simulink subsystem "RT_BladeElementForces"  (R2025a)
settings: Solver=VariableStepAuto  StartTime=0.0  StopTime=10.0  RelTol=1e-3
undefined symbols (not defined in the file): RT_AirDensity_P, RT_BEDistFromEffSta_A, RT_NondimRadialDisRef_P, RT_NumberOfBlades_P, RT_RotorRadius_P, RT_SigmaAvgUH60_P, RT_SonicVel_P, RT_TaperedRatio_P, RT_Weight_P
settings Model: DataDictionary=Rotor.sldd  EnableAccessToBaseWorkspace=off  Creator=Admin  LastModifiedBy=Admin

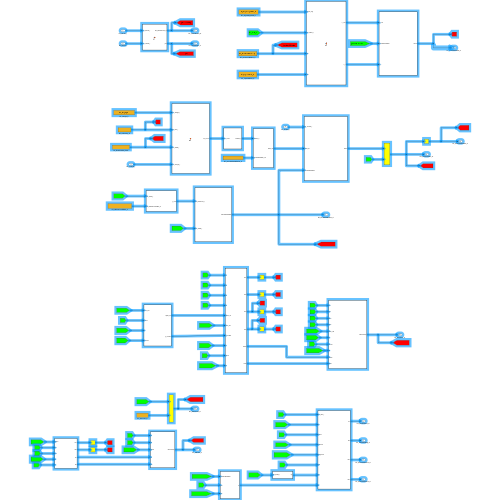
[thumbnail: Simulink's stored preview of the top-level diagram]
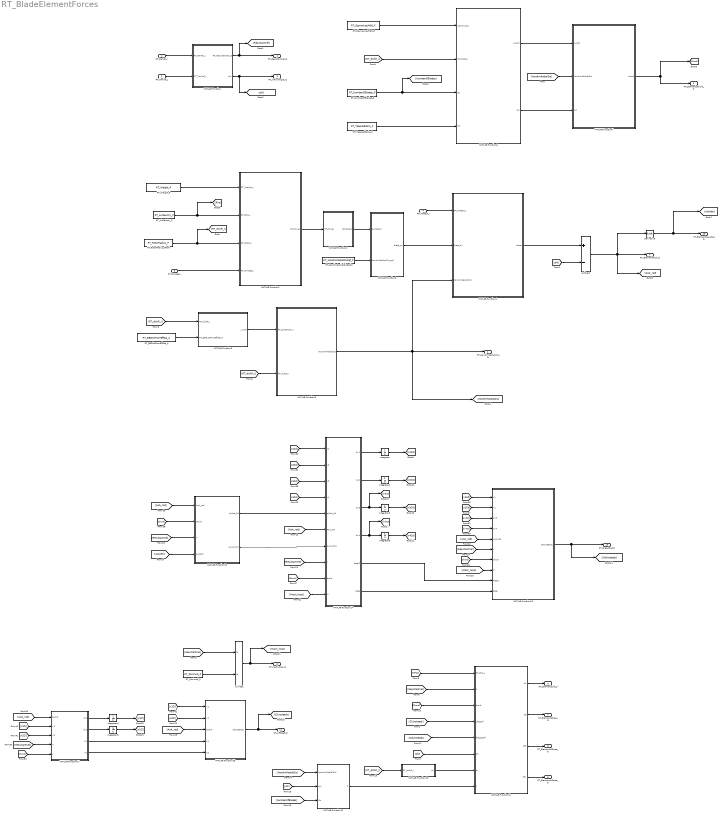
== system RT_BladeElementForces ==
  "RT_PerVel_I " : Inport
  RT_TanVel_I : Inport  Port=2
  RT_Omega_I : Inport  Port=3
  RT_Theta0_I : Inport  Port=4
  Derivative : Derivative
  Divide1 : Product  Inputs=*/
  Integrator{,1..5} (6 alike) : Integrator
  MATLAB Function : MATLAB Function  TreatAsAtomicUnit=on
  MATLAB Function1 : MATLAB Function  TreatAsAtomicUnit=on
  MATLAB Function10 : MATLAB Function  TreatAsAtomicUnit=on
  MATLAB Function11 : MATLAB Function  TreatAsAtomicUnit=on
  MATLAB Function12 : MATLAB Function  TreatAsAtomicUnit=on
  MATLAB Function13 : MATLAB Function  TreatAsAtomicUnit=on
  MATLAB Function14 : MATLAB Function  TreatAsAtomicUnit=on
  MATLAB Function15 : MATLAB Function  TreatAsAtomicUnit=on
  MATLAB Function17 : MATLAB Function  TreatAsAtomicUnit=on
  MATLAB Function18 : MATLAB Function  TreatAsAtomicUnit=on
  MATLAB Function2 : MATLAB Function  TreatAsAtomicUnit=on
  MATLAB Function3 : MATLAB Function  TreatAsAtomicUnit=on
  MATLAB Function4 : MATLAB Function  TreatAsAtomicUnit=on
  MATLAB Function6 : MATLAB Function  TreatAsAtomicUnit=on
  MATLAB Function7 : MATLAB Function  TreatAsAtomicUnit=on
  MATLAB Function8 : MATLAB Function  TreatAsAtomicUnit=on
  MATLAB Function9 : MATLAB Function  TreatAsAtomicUnit=on
  RT_AirDensity_P : Constant  Value=RT_AirDensity_P
  RT_BEDistFromEffSta_A : Constant  Value=RT_BEDistFromEffSta_A
  RT_NondimRadialDisRef_P : Constant  Value=RT_NondimRadialDisRef_P
  RT_NumberOfBlades_P : Constant  Value=RT_NumberOfBlades_P
  RT_RotorRadius_Ptant : Constant  Value=RT_RotorRadius_P
  RT_SigmaAvgUH60_P : Constant  Value=RT_SigmaAvgUH60_P
  RT_SonicVel_P : Constant  Value=RT_SonicVel_P
  RT_TaperedRatio_P : Constant  Value=RT_TaperedRatio_P
  RT_Weight_P : Constant  Value=RT_Weight_P
  Subtract : Sum  Inputs=+-
  RT_NondimRadialDis_O : Outport
  RT_ResultantVel_O : Outport  Port=2
  RT_InflowAngle_O : Outport  Port=3
  RT_ElementsAoA_O : Outport  Port=4
  RT_ElementsChord_O : Outport  Port=5
  RT_ElementsLift_O : Outport  Port=6
  RT_ElementsDrag_O : Outport  Port=7
  RT_ElementsZForce_O : Outport  Port=8
  RT_ElementsXForce_O : Outport  Port=9
  RT_DragCoef_O : Outport  Port=10
  RT_LiftCoef_O : Outport  Port=11
  RT_MachLocal_O : Outport  Port=12
  RT_ElementsAoAdot_O : Outport  Port=13
  wires:
  MATLAB Function12/1(F) -> MATLAB Function11/8(F)
  [Mach_local] -> MATLAB Function14/10(M)
  MATLAB Function17/1(dx1) -> Integrator4/1
  Integrator2/1 -> [x3Cd]
  [Chord] -> MATLAB Function15/7(chord)
  Integrator4/1 -> [x1Cl]
  [Rho] -> MATLAB Function11/1(RT_Rho_I)
  [Chord] -> MATLAB Function17/5(c)
  [CdUnsteady] -> MATLAB Function11/5(DragCoef)
  [AoA_rad] -> MATLAB Function13/1(AoA_rad)
  Subtract/1 -> Derivative/1, RT_ElementsAoA_O/1, [AoA_rad]
  [ResultantVel] -> MATLAB Function14/8(V)
  Derivative/1 -> [AoAdot], RT_ElementsAoAdot_O/1
  [ResultantVel] -> MATLAB Function15/6(V)
  MATLAB Function1/1(CT_hover) -> MATLAB Function2/1(CT_hover)
  [phi] -> MATLAB Function12/2(phi)
  MATLAB Function14/3(dx3) -> [dx3Cd], Integrator2/1
  MATLAB Function6/1(c_root) -> MATLAB Function7/1(c_root)
  RT_Theta0_I/1 -> MATLAB Function4/1(RT_Theta0_I)
  MATLAB Function11/3(dFz) -> RT_ElementsZForce_O/1
  MATLAB Function3/1(theta_tw) -> MATLAB Function4/2(theta_tw)
  MATLAB Function4/1(theta) -> Subtract/1
  MATLAB Function13/1(alpha_34) -> MATLAB Function14/5(alpha_34)
  RT_NondimRadialDisRef_P/1 -> MATLAB Function3/2(NondimRadialDis_ref)
  [Chord] -> MATLAB Function14/9(chord)
  [AoA_rad] -> MATLAB Function18/3(alpha)
  RT_Omega_I/1 -> MATLAB Function1/4(RT_Omega_I)
  MATLAB Function17/3(K1) -> MATLAB Function18/4(K1)
  MATLAB Function10/1(dy) -> MATLAB Function11/7(dy)
  [x2Cd] -> MATLAB Function14/2(x2)
  [Mach_local] -> MATLAB Function15/8(M)
  MATLAB Function11/4(dFx) -> RT_ElementsXForce_O/1
  MATLAB Function6/2(t_c) -> MATLAB Function7/3(t_c)
  [x2Cl] -> MATLAB Function18/2(x2)
  MATLAB Function/1(RT_ResultantVel_O) -> [ResultantVel], RT_ResultantVel_O/1
  [phi] -> Subtract/2
  MATLAB Function17/2(dx2) -> Integrator5/1
  MATLAB Function14/4(dx4) -> [dx4Cd], Integrator3/1
  [dx3Cd] -> MATLAB Function15/3(dx3)
  [RT_diskR_I] -> MATLAB Function6/2(RT_diskR_I)
  Integrator1/1 -> [x2Cd]
  MATLAB Function14/5(beta2) -> MATLAB Function15/9(beta2)
  RT_TaperedRatio_P/1 -> MATLAB Function6/4(TR)
  [NondimRadialDis] -> MATLAB Function12/1(NondimRadialDis)
  [dx4Cd] -> MATLAB Function15/4(dx4)
  Divide1/1 -> [Mach_local], RT_MachLocal_O/1
  [AoAdot] -> MATLAB Function13/4(AoAdot)
  [x2Cd] -> MATLAB Function15/2(x2)
  [x1Cd] -> MATLAB Function15/1(x1)
  MATLAB Function8/1(NondimRadialDis) -> MATLAB Function4/3(NondimRadialDis), [NondimRadialDis], RT_NondimRadialDis_O/1
  [ResultantVel] -> MATLAB Function17/4(V)
  Integrator3/1 -> [x4Cd]
  [RT_diskR_I] -> MATLAB Function8/2(RT_diskR_I)
  [ResultantVel] -> MATLAB Function13/3(V)
  [x1Cl] -> MATLAB Function17/2(x1)
  MATLAB Function11/1(dL) -> RT_ElementsLift_O/1
  [RT_diskR_I] -> MATLAB Function10/1(RT_diskR_I)
  RT_SigmaAvgUH60_P/1 -> MATLAB Function6/1(sigma_avg)
  "RT_PerVel_I "/1 -> MATLAB Function/1(RT_PerVel_I)
  [x3Cd] -> MATLAB Function14/3(x3)
  MATLAB Function14/2(dx2) -> Integrator1/1
  Integrator5/1 -> [x2Cl]
  [Chord] -> MATLAB Function11/3(chord)
  [x1Cd] -> MATLAB Function14/1(x1)
  MATLAB Function18/1(ClUnsteady) -> RT_LiftCoef_O/1, [ClUnsteady]
  MATLAB Function15/1(CdUnsteady) -> RT_DragCoef_O/1, [CdUnsteady]
  [NumberOfBlades] -> MATLAB Function12/3(Nb)
  [Chord] -> MATLAB Function13/2(chord)
  Integrator/1 -> [x1Cd]
  RT_RotorRadius_Ptant/1 -> [RT_diskR_I], MATLAB Function1/3(RT_diskR_I)
  MATLAB Function/2(phi) -> [phi], RT_InflowAngle_O/1
  [ClUnsteady] -> MATLAB Function11/4(LiftCoef)
  RT_BEDistFromEffSta_A/1 -> MATLAB Function9/2(RT_BEDistFromEffSta_A)
  RT_AirDensity_P/1 -> [Rho], MATLAB Function1/2(RT_Rho_I)
  RT_TanVel_I/1 -> MATLAB Function/2(RT_TanVel_I)
  [x4Cd] -> MATLAB Function14/4(x4)
  [NondimRadialDis] -> MATLAB Function7/2(NondimRadialDis)
  RT_Weight_P/1 -> MATLAB Function1/1(RT_Weight_I)
  MATLAB Function13/2(q_nondim) -> MATLAB Function14/7(q_nondim)
  [x2Cl] -> MATLAB Function17/3(x2)
  RT_SonicVel_P/1 -> Divide1/2
  MATLAB Function11/2(dD) -> RT_ElementsDrag_O/1
  [x1Cl] -> MATLAB Function18/1(x1)
  [AoA_rad] -> MATLAB Function15/5(AoA_rad)
  [ResultantVel] -> Divide1/1
  [RT_diskR_I] -> MATLAB Function9/1(RT_diskR_I)
  MATLAB Function17/4(K2) -> MATLAB Function18/5(K2)
  [ResultantVel] -> MATLAB Function11/2(U)
  [phi] -> MATLAB Function11/6(phi)
  RT_NumberOfBlades_P/1 -> [NumberOfBlades], MATLAB Function6/3(Nb)
  MATLAB Function14/6(beta) -> MATLAB Function15/10(beta)
  MATLAB Function14/1(dx1) -> Integrator/1
  [AoA_rad] -> MATLAB Function14/6(AoA_rad)
  MATLAB Function9/1(y_mat) -> MATLAB Function8/1(RT_DistanceY_I)
  MATLAB Function2/1(lambda_h) -> MATLAB Function3/1(lambda_h)
  [AoA_rad] -> MATLAB Function17/1(alpha)
  MATLAB Function7/1(chord) -> RT_ElementsChord_O/1, [Chord]

== matlab function RT_BladeElementForces/MATLAB Function10 ==
  data: RT_diskR_I input; dy output
function dy = fcn(RT_diskR_I)

r0 = 0.05;
N  = 20;
dy = RT_diskR_I * (1 - r0) / N;

== matlab function RT_BladeElementForces/MATLAB Function11 ==
  data: RT_Rho_I input; dL output; U input; chord input; LiftCoef input; DragCoef input; phi input; dy input; dD output; dFz output; dFx output; F input
function [dL, dD, dFz, dFx] = fcn(RT_Rho_I, U, chord, LiftCoef, DragCoef, phi, dy, F)

q    = 0.5 .* RT_Rho_I .* U.^2 .* chord .* dy;

dL   = q .* LiftCoef;
dD   = q .* DragCoef;

dFz  = (dL .* cos(phi) - dD .* sin(phi)) .* F;
dFx  = (dL .* sin(phi) + dD .* cos(phi)) .* F;

== matlab function RT_BladeElementForces/MATLAB Function12 ==
  data: NondimRadialDis input; F output; phi input; Nb input
function F = fcn(NondimRadialDis, phi, Nb)

r   = NondimRadialDis;
phi_safe = abs(phi) + 1e-6;

% f_tip — Eq. 3.121
f_tip  = (Nb/2) .* (1 - r) ./ (r .* phi_safe);

% f_root — Eq. 3.127
f_root = (Nb/2) .* r ./ ((1 - r) .* phi_safe);

% F_tip và F_root riêng — Eq. 3.120
F_tip  = (2/pi) .* acos(min(exp(-f_tip),  1.0));
F_root = (2/pi) .* acos(min(exp(-f_root), 1.0));

% Kết hợp — Eq. 3.128
F = F_tip .* F_root;

== matlab function RT_BladeElementForces/MATLAB Function13 ==
  data: AoA_rad input; alpha_34 output; chord input; V input; AoAdot input; q_nondim output
function [alpha_34, q_nondim] = fcn(AoA_rad, chord, V, AoAdot)
%% BLOCK 1 — AoA tại điểm 3/4 chord (alpha_34)
% =========================================================
% NGUỒN GỐC LÝ THUYẾT:
%   Leishman & Nguyen (1990) AIAA Journal, Vol.28 No.5
%   Eq. sau Eq.(17): alpha_34 = alpha(t) + q(t)/2
%
%   Trong đó q là NONDIMENSIONAL pitch rate:
%   q_nondim = q_actual * c / V = (dtheta/dt) * c / V
%
%   Ý nghĩa của alpha_34:
%   Theodorsen (1935) chứng minh rằng với thin airfoil theory,
%   điểm 3/4 chord là "aerodynamic center" cho unsteady flow.
%   Đây là điểm mà downwash boundary condition phải được thỏa
%   mãn để cho kết quả chính xác nhất về unsteady lift.
%
%   Khi cánh có pitch rate q_actual (rad/s):
%   - Điểm 1/4 chord: AoA = alpha (geometric)
%   - Điểm 3/4 chord: AoA = alpha + q_actual*(c/2)/V
%     vì điểm 3/4 chord cách điểm pitch một khoảng c/2,
%     tốc độ pháp tuyến thêm = q_actual * (c/2)
%     góc thêm = q_actual*(c/2)/V = q_nondim/2
%
%   Tại sao cần alpha_34 thay vì alpha thông thường?
%   - Dùng alpha thông thường → bỏ qua pitch rate effect
%   - Với hover steady (q=0): alpha_34 = alpha → không sai
%   - Với maneuver (q≠0): alpha_34 ≠ alpha → cần thiết
%
% PITCH RATE q_nondim = theta_dot*c/V + beta_d*c/V:
%
%   Thành phần 1 — theta_dot (dθ₀/dt):
%   Khi pilot thay đổi collective θ₀(t) → cánh xoay quanh
%   pitch axis với tốc độ theta_dot = dθ₀/dt (rad/s).
%   Lấy từ: Transfer Function 100s/(s+100) sau RT_Theta0_I
%   (lọc high-pass để loại noise, giữ thay đổi thực)
%
%   Thành phần 2 — beta_d (dβ/dt):
%   Khi cánh flap với tốc độ beta_d (rad/s), chuyển động
%   vẫy lên/xuống tương đương với pitch rate tại section.
%   Lấy từ: inport 7 của Relative Wind Velocity block
%   (đã có sẵn, không cần lấy đạo hàm thêm)
%
%   Tại sao KHÔNG cộng azimuth effect vào q?
%   AoA thay đổi theo ψ (azimuth) do velocity field thay đổi
%   đã được capture hoàn toàn trong:
%   AoA = theta - phi, với phi = atan2(U_P, U_T)
%   U_P, U_T đã bao gồm tất cả hiệu ứng azimuth qua psi input
%   của Relative Wind Velocity block.
%   q trong Leishman chỉ là MECHANICAL pitch rate của blade,
%   không phải rate of change of AoA due to velocity field.
%
% INPUTS:
%   AoA_rad   [20x1] : góc tấn geometric (rad) = theta(r) - phi
%                      thay đổi theo r̄, ψ, và t
%                      từ Sum block (theta - phi)
%   chord     [20x1] : chord tại từng element (m) = c(r̄)
%                      từ Block chord distribution
%                      = c_root*(1 - t_c*r_bar) với TR=3/7
%   V         [20x1] : vận tốc tổng hợp (m/s) = sqrt(U_P²+U_T²)
%                      từ Block U/phi (ResultantVel)
%                      dùng để nondimensionalize q
%   theta_dot [1x1]  : dθ₀/dt (rad/s) — collective pitch rate
%                      từ Transfer Fcn sau RT_Theta0_I
%                      = 0 khi hover steady
%   beta_d    [1x1]  : dβ/dt (rad/s) — flapping rate
%                      từ inport 7 của model
%                      = 0 khi không có flapping
%
% OUTPUT:
%   alpha_34  [20x1] : AoA tại điểm 3/4 chord (rad)
%                      = AoA_rad khi q = 0
%                      được dùng làm input cho Block 2 (derivatives)
%                      thay thế cho AoA_rad trong circulatory states
%
% NGUỒN: Leishman & Nguyen (1990) AIAA J. Vol.28 No.5, p.839
%        Eq. sau Eq.(17); Theodorsen (1935) NACA Rept.496
% =========================================================

%% Bước 1 — Tổng hợp pitch rate vật lý (rad/s)
% q_actual = tổng đóng góp cơ học vào pitch rate của blade section
% Không bao gồm azimuth effect (đã có trong AoA = theta - phi)
q_actual = AoAdot;   % [1x1] scalar (rad/s)

%% Bước 2 — Nondimensionalize: q_nondim = q_actual * c / V
% Chuẩn hóa theo Leishman & Nguyen (1990) Nomenclature: q = αc/V
% [20x1]: mỗi element có chord và V khác nhau → q_nondim khác nhau
q_nondim = q_actual .* chord ./ max(V, 1e-4);
% max(V, 1e-4): tránh chia 0 khi rotor dừng (V → 0)

%% Bước 3 — AoA tại 3/4 chord
% alpha_34 = alpha + q_nondim/2
% Eq. sau Eq.(17) trong Leishman & Nguyen (1990)
% Hệ số 1/2: khoảng cách từ điểm pitch đến 3/4 chord = c/2
%            nondim bởi c: (c/2)/c = 1/2
alpha_34 = AoA_rad + q_nondim ./ 2;

end

== matlab function RT_BladeElementForces/MATLAB Function14 ==
  data: x1 input; dx1 output; x2 input; x3 input; x4 input; alpha_34 input; AoA_rad input; q_nondim input; V input; chord input; M input; dx2 output; dx3 output; dx4 output; beta2 output; beta output
function [dx1, dx2, dx3, dx4, beta2, beta] = fcn(x1, x2, x3, x4, alpha_34, AoA_rad, q_nondim, V, chord, M)
%% BLOCK 2 v2 — Đạo hàm 4 ODE states
% =========================================================
% NGUỒN: Leishman & Nguyen (1990) AIAA J. Vol.28 No.5
%
% 4 STATES ĐẦY ĐỦ CHO Cn:
%   x1, x2 — Circulatory từ alpha     [Eq.17]
%   x3     — Noncirculatory từ alpha  [Eq.19]
%   x4     — Noncirculatory từ q      [Appendix A, Eq.A3]
%
% TẠI SAO CẦN x4?
%   D matrix của state-space (trang 4 paper):
%   Cn = C*x + D*{alpha, q}
%   D(1,:) = [4/M, 1/M]
%   → Cn có 2 direct feedthrough terms:
%     4/M * alpha  ← đến từ ẋ3 (x3 state)
%     1/M * q      ← đến từ ẋ4 (x4 state)
%   Nếu bỏ x4 → thiếu thành phần Cn noncirculatory từ q
%
% STATE x4 — Noncirculatory từ q (Appendix A, Eq.A3):
%   ẋ4 = q(t) - (1/(K_q*T_I))*x4 = q(t) + a44*x4
%
%   K_q(M) = [(1-M) + 2π*β*M²*(A1*b1+A2*b2)]⁻¹
%   Giảm 25% theo thực nghiệm: K_q_actual = 0.75*K_q_theory
%
%   C_N^I_q = (1/M)*ẋ4   [Eq.A4]
%
%   Ý nghĩa: apparent mass từ pitch rate
%   Khi cánh xoay nhanh (q lớn) → gia tốc khối khí quanh cánh
%   → lực pháp tuyến tức thì tỷ lệ (1/M)*q
%   Decay theo K_q*T_I tương tự x3
%
% INPUTS:
%   x1,x2    [4x20] : circulatory states — từ Integrators 1,2
%   x3       [4x20] : noncirculatory alpha state — từ Integrator 3
%   x4       [4x20] : noncirculatory q state — từ Integrator 4
%   alpha_34 [4x20] : AoA tại 3/4 chord (rad) — từ Block 1
%   AoA_rad  [4x20] : AoA geometric (rad) = theta - phi
%   q_nondim [4x20] : nondimensional pitch rate = q_actual*c/V
%                     = (theta_dot + beta_d)*chord/V
%   V        [4x20] : vận tốc tổng hợp (m/s)
%   chord    [4x20] : chord tại element (m)
%   M        [4x20] : Mach cục bộ
%
% OUTPUTS:
%   dx1 [4x20] → Integrator 1 (IC=zeros(20,1))
%   dx2 [4x20] → Integrator 2 (IC=zeros(20,1))
%   dx3 [4x20] → Integrator 3 (IC=zeros(20,1))
%   dx4 [4x20] → Integrator 4 (IC=zeros(20,1))
%
% NGUỒN: Leishman & Nguyen (1990)
%   x1,x2: Eq.(17); x3: Eq.(19); x4: Appendix A Eq.(A3)
% =========================================================

%% Hằng số Beddoes — Leishman & Nguyen (1990) trang 4
A1 = 0.3;   b1 = 0.14;
A2 = 0.7;   b2 = 0.53;
a_sound = 340;   % m/s

%% Prandtl-Glauert
beta2 = max(1 - M.^2, 0.01);
beta  = sqrt(beta2);

%% Hệ số chuyển đổi reduced time → real time
coeff = (2 .* V ./ max(chord, 1e-4)) .* beta2;

%% ── x1, x2: Circulatory từ alpha (Eq.17) ──────────────────────
% Input: alpha_34 = alpha + q_nondim/2 (AoA tại 3/4 chord)
% b1=0.14 (chậm), b2=0.53 (nhanh) — Beddoes constants
dx1 = -b1 .* coeff .* x1 + alpha_34;
dx2 = -b2 .* coeff .* x2 + alpha_34;

%% ── K_alpha(M) cho x3 — Eq. sau Eq.(16) ───────────────────────
% K_alpha_theory = [(1-M) + π*β*M²*(A1*b1+A2*b2)]⁻¹
% Giảm 25%: K_alpha_actual = 0.75*K_alpha_theory
K_alpha_theory = 1 ./ ((1-M) + pi.*beta.*M.^2.*(A1.*b1+A2.*b2));
K_alpha = 0.75 .* K_alpha_theory;

%% ── T_I = c/a — Acoustic travel time ──────────────────────────
% Dùng a_sound (tốc độ âm), KHÔNG phải V
Ti = chord ./ a_sound;

%% ── x3: Noncirculatory từ alpha (Eq.19) ───────────────────────
% ẋ3 = alpha + a33*x3, với a33 = -1/(K_alpha*T_I)
a33 = -1 ./ (K_alpha .* Ti);
dx3 = a33 .* x3 + AoA_rad;

%% ── K_q(M) cho x4 — Appendix A, Eq.(A2) ──────────────────────
% K_q(M) = [(1-M) + 2π*β*M²*(A1*b1+A2*b2)]⁻¹
% Từ paper: K_q có cùng dạng K_alpha nhưng với hệ số 2π thay π
% Giảm 25% theo thực nghiệm tương tự K_alpha
K_q_theory = 1 ./ ((1-M) + 2*pi.*beta.*M.^2.*(A1.*b1+A2.*b2));
K_q = 0.75 .* K_q_theory;

%% ── x4: Noncirculatory từ q (Appendix A, Eq.A3) ───────────────
% ẋ4 = q(t) - (1/(K_q*T_I))*x4 = q(t) + a44*x4
% Input: q_nondim (đã nondimensionalize = q_actual*c/V)
% a44 = -1/(K_q*T_I) — eigenvalue âm, hệ ổn định
a44 = -1 ./ (K_q .* Ti);
dx4 = a44 .* x4 + q_nondim;

end

== matlab function RT_BladeElementForces/MATLAB Function15 ==
  data: x1 input; x2 input; dx3 input; dx4 input; AoA_rad input; V input; chord input; M input; beta2 input; beta input; CdUnsteady output
function CdUnsteady = fcn(x1, x2, dx3, dx4, AoA_rad, V, chord, M, beta2, beta)
%% BLOCK 3 v2 — Cn(t) và CdUnsteady đầy đủ theo paper 1990
% =========================================================
% NGUỒN: Leishman & Nguyen (1990) AIAA J. Vol.28 No.5
%
% CẤU TRÚC Cn ĐẦY ĐỦ — Eq.(21):
%   Cn(t) = C_N^C(t) + C_N^I_alpha(t) + C_N^I_q(t)
%
%   C_N^C      : Eq.(18) — circulatory, từ x1,x2
%   C_N^I_alpha: Eq.(20) — noncirculatory từ alpha, từ ẋ3
%   C_N^I_q    : Eq.(A4) — noncirculatory từ q, từ ẋ4
%
% TẠI SAO CÓ 3 THÀNH PHẦN?
%
%   C_N^C — Shed wake (circulatory):
%   Khi alpha thay đổi → circulation Γ thay đổi → wake vortex
%   bị shed từ trailing edge → wake downwash làm giảm effective AoA
%   → Cn build up chậm theo Wagner function
%   Phụ thuộc LỊCH SỬ alpha qua x1, x2
%
%   C_N^I_alpha — Apparent mass từ alpha (noncirculatory):
%   Khi alpha thay đổi nhanh → phải gia tốc khối khí quanh cánh
%   → lực quán tính tức thì ∝ dα/dt
%   Từ piston theory: initial value = 4/M * dα/dt * (c/2V)
%   Decay theo acoustic travel time K_alpha*T_I = K_alpha*c/a
%   Phụ thuộc TỐC ĐỘ THAY ĐỔI alpha, không phải alpha
%
%   C_N^I_q — Apparent mass từ pitch rate (noncirculatory):
%   Khi q thay đổi → gia tốc góc thêm → lực quán tính tức thì
%   Initial value = 1/M * dq/dt * (c/2V)
%   Decay tương tự C_N^I_alpha nhưng với K_q thay K_alpha
%   Phụ thuộc TỐC ĐỘ THAY ĐỔI q
%
% INPUTS:
%   x1, x2   [4x20] : circulatory states — từ Integrators 1,2
%   x3       [4x20] : noncirculatory alpha state — từ Integrator 3
%   x4       [4x20] : noncirculatory q state — từ Integrator 4
%   AoA_rad  [4x20] : góc tấn geometric (rad) = theta - phi
%   q_nondim [4x20] : nondimensional pitch rate = q_actual*c/V
%                     = (theta_dot + beta_d)*chord/V
%   V        [4x20] : vận tốc tổng hợp (m/s)
%   chord    [4x20] : chord tại element (m)
%   M        [4x20] : Mach cục bộ = V/340
%
% OUTPUTS:
%   Cn       [4x20] : normal force coeff unsteady — Eq.(21)
%   CdUnsteady [4x20] : drag coeff unsteady — Eq.(24) + Cd0
%
% NGUỒN: Leishman & Nguyen (1990)
%   Cn_c:        Eq.(18)
%   Cn_nc_alpha: Eq.(20)
%   Cn_nc_q:     Appendix A, Eq.(A4)
%   alpha_E:     Eq.(22)
%   Cc:          Eq.(23)
%   Cd:          Eq.(24)
% =========================================================

%% Hằng số Beddoes
A1 = 0.3;   b1 = 0.14;
A2 = 0.7;   b2 = 0.53;

%% ── BƯỚC 1: Cn circulatory — Eq.(18) ──────────────────────────
% C_N^C = (2π/β)*(2V/c)*β²*(A1*b1*x1 + A2*b2*x2)
%
% Giải thích từng nhân tử:
% (2π/β)    : lift curve slope compressible (Prandtl-Glauert)
%              incompressible 2π → compressible 2π/β
% (2V/c)*β² : chuyển reduced time ds/dt=2V/c, scale β² cho poles
% A1*b1*x1  : đóng góp của state x1 (ký ức dài, b1=0.14)
% A2*b2*x2  : đóng góp của state x2 (ký ức ngắn, b2=0.53)
% Tổng: reconstruction của Duhamel integral qua 2 ODE states
coeff_c = (2*pi./beta) .* (2.*V./max(chord,1e-4)) .* beta2;
Cn_c = coeff_c .* (A1.*b1.*x1 + A2.*b2.*x2);

%% ── BƯỚC 2: Cn noncirculatory từ alpha — Eq.(20) ──────────────
% C_N^I_alpha = (4/M) * ẋ3
%
% Tính ẋ3 = a33*x3 + AoA_rad (từ Eq.19, giống Block 2)
% (4/M): hệ số piston theory cho noncirculatory từ alpha
%        tại M thấp (hover): 4/M lớn → apparent mass đáng kể
Cn_nc_alpha = (4./max(M,0.01)).*dx3;   % Eq.(20)

%% ── BƯỚC 3: Cn noncirculatory từ q — Appendix A, Eq.(A4) ──────
% C_N^I_q = (1/M) * ẋ4
%
% Tính ẋ4 = a44*x4 + q_nondim (từ Eq.A3, giống Block 2)
% (1/M): hệ số piston theory cho noncirculatory từ q
%        nhỏ hơn 4/M của alpha term
Cn_nc_q = (1./max(M,0.01)).*dx4;   % Eq.(A4)

%% ── BƯỚC 4: Cn total — Eq.(21) ────────────────────────────────
% Cộng tuyến tính 3 thành phần
% Cn_c:       lớn nhất, phụ thuộc lịch sử alpha
% Cn_nc_alpha: trung bình, phụ thuộc dα/dt
% Cn_nc_q:    nhỏ nhất, phụ thuộc dq/dt
Cn = Cn_c + Cn_nc_alpha + Cn_nc_q;

%% ── BƯỚC 5: alpha_E — Effective AoA — Eq.(22) ─────────────────
% alpha_E = β²*(2V/c)*(A1*b1*x1 + A2*b2*x2)
%
% alpha_E là AoA mà airfoil "thực sự cảm nhận" sau Wagner lag
% Khi step change mới: x1,x2 ≈ 0 → alpha_E ≈ 0 (chưa build up)
% Khi steady: x1→alpha/(b1*coeff_s), x2→alpha/(b2*coeff_s)
%             → alpha_E → alpha (full build up)
% alpha_E chỉ phụ thuộc circulatory states (x1,x2)
% KHÔNG bao gồm noncirculatory (x3,x4) vì Cc = leading edge suction
% chỉ đến từ circulatory loading (Eq.22 paper)
alpha_E = beta2.*(2.*V./max(chord,1e-4)).*(A1.*b1.*x1 + A2.*b2.*x2);

%% ── BƯỚC 6: Cc chord force — Eq.(23) ──────────────────────────
% Cc = (2π/β) * alpha_E²
%
% Leading edge suction force — kéo cánh về phía trước
% Tỷ lệ BÌNH PHƯƠNG alpha_E → nonlinear
% Giải thích: Cc = ∫ Cp * cos(surface_angle) ds
%             ≈ π * Γ²/V² ∝ alpha_E²
% Khi alpha_E lớn (steady state) → Cc lớn → giảm Cd (suction kéo)
% Khi alpha_E nhỏ (unsteady initial) → Cd tăng (mất suction)
% Đây là lý do Cd tăng trong ramp forcing (Fig.9 paper)
Cc = (2*pi./beta).*alpha_E.^2;

%% ── BƯỚC 7: Cd0 — Viscous drag từ C81 ─────────────────────────
% Cd0 = viscous (skin friction) drag tại alpha=0
% Không đổi theo unsteady effects (Leishman §8.15.7):
% "viscous shear stress drag is nominally constant below stall"
% Cộng thêm riêng vào Eq.(24) vì Eq.(24) chỉ tính pressure drag
% Lý tưởng: Cd0 = F_Cd(zeros(20,1), M_local) từ C81 table
Cd0 = 0.009.*ones(size(M));   % NACA 0012 tại alpha=0, M=0.3-0.5
% TODO: đổi thành F_Cd(zeros(20,1), M) khi có workspace access

%% ── BƯỚC 8: CdUnsteady — Eq.(24) + Cd0 ─────────────────────────
% Eq.(24): C_D = C_N*sin(α) - C_C*cos(α)   ← pressure drag only
%
% Giải thích hình học (Fig.4 paper):
% Cn hướng vuông góc chord → hình chiếu lên drag: Cn*sin(α)
% Cc hướng dọc chord (LE direction) → hình chiếu lên drag: -Cc*cos(α)
% Tổng: C_D_pressure = Cn*sin(α) - Cc*cos(α)
%
% Ý nghĩa unsteady:
% Khi Cc giảm (mất leading edge suction) → Cd tăng
% Đây capture được "leading edge suction analog" trong unsteady flow
% Với Cn tăng (apparent mass) và Cc giảm → Cd tăng mạnh
% Phù hợp với Fig.9 paper: Cd tăng với ramp rate
CdUnsteady = Cn.*sin(AoA_rad) - Cc.*cos(AoA_rad) + Cd0;
CdUnsteady = max(CdUnsteady, 0.005);   % clamp: Cd không âm

end

== matlab function RT_BladeElementForces/MATLAB Function17 ==
  data: alpha input; dx1 output; x1 input; x2 input; V input; c input; dx2 output; K1 output; K2 output
function [dx1, dx2, K1, K2] = aero_states(alpha, x1, x2, V, c)
% ============================================================
% UNSTEADY AERODYNAMIC STATE MODEL (WAGNER → STATE-SPACE)
% ============================================================
%
% THEORY:
%
% Original problem:
% Lift depends on past history (wake memory):
%
%   Cl(t) = ∫ alpha_dot(τ) * phi(t-τ) dτ
%
% where phi(s) = Wagner function
%
% This is a convolution → expensive in simulation.
%
% SOLUTION:
% Use Jones approximation:
%
%   phi(s) ≈ 1 - A1*e^(-b1*s) - A2*e^(-b2*s)
%
% This allows conversion into ODE form:
%
%   x1_dot = x2
%   x2_dot = -a1*x1 - a2*x2 + alpha
%
% This is EXACTLY the finite-state model introduced by:
% → Friedmann (1985)
%
% So this block = wake memory dynamics
%
% ============================================================

% Reduced velocity terms
K1 = 2 .* V ./ c;
K2 = (2 .* V ./ c).^2;

% Coefficients (Jones approximation)
a1 = 0.01375 .* K2;
a2 = 0.3455  .* K1;

% State equations (element-wise)
dx1 = x2;

dx2 = -a1 .* x1 ...
      -a2 .* x2 ...
      + alpha;


end

== matlab function RT_BladeElementForces/MATLAB Function18 ==
  data: x1 input; ClUnsteady output; x2 input; alpha input; K1 input; K2 input
function ClUnsteady = compute_Cl(x1, x2, alpha, K1, K2)
% ============================================================
% UNSTEADY LIFT COEFFICIENT COMPUTATION
% ============================================================
%
% THEORY:
%
% Lift = Circulatory + Non-circulatory
%
% Circulatory:
%   Comes from wake (depends on x1, x2)
%
% Non-circulatory:
%   Instantaneous response to alpha
%
% Final model (Leishman Eq. 8.113):
%
%   Cl = 2π*(C1*x1 + C2*x2) + π/2 * alpha
%
% IMPORTANT:
% π/2 * alpha term exists because:
% Wagner function has non-zero initial value:
%   phi(0) ≠ 0
%
% This ensures equivalence with:
% - Theodorsen solution
% - Wagner solution
%
% ============================================================


ClUnsteady = 2*pi*( ...
      0.006825 .* K2 .* x1 + ...
      0.10805  .* K1 .* x2 ) ...
     + (pi/2) .* alpha;


end

== matlab function RT_BladeElementForces/MATLAB Function1 ==
  data: RT_Weight_I input; CT_hover output; RT_Rho_I input; RT_diskR_I input; RT_Omega_I input
function CT_hover = fcn(RT_Weight_I, RT_Rho_I, RT_diskR_I, RT_Omega_I)

CT_hover = (RT_Weight_I) / ...
           (RT_Rho_I * pi * RT_diskR_I^2 * (RT_Omega_I * RT_diskR_I)^2);

== matlab function RT_BladeElementForces/MATLAB Function ==
  data: RT_PerVel_I input; RT_ResultantVel_O output; RT_TanVel_I input; phi output
function [RT_ResultantVel_O, phi] = fcn(RT_PerVel_I, RT_TanVel_I)

RT_ResultantVel_O = sqrt(RT_PerVel_I.^2 + RT_TanVel_I.^2);
phi               = atan2(RT_PerVel_I, RT_TanVel_I);

== matlab function RT_BladeElementForces/MATLAB Function2 ==
  data: CT_hover input; lambda_h output
function lambda_h = fcn(CT_hover)

lambda_h = sqrt(CT_hover / 2);

== matlab function RT_BladeElementForces/MATLAB Function3 ==
  data: lambda_h input; theta_tw output; NondimRadialDis_ref input
function theta_tw = fcn(lambda_h, NondimRadialDis_ref)

theta_tw = -lambda_h / NondimRadialDis_ref^2;

== matlab function RT_BladeElementForces/MATLAB Function4 ==
  data: RT_Theta0_I input; theta output; theta_tw input; NondimRadialDis input
function theta = fcn(RT_Theta0_I, theta_tw, NondimRadialDis)

theta = RT_Theta0_I + theta_tw .* NondimRadialDis;

== matlab function RT_BladeElementForces/MATLAB Function6 ==
  data: sigma_avg input; c_root output; RT_diskR_I input; Nb input; TR input; t_c output
function [c_root, t_c] = fcn(sigma_avg, RT_diskR_I, Nb, TR)

t_c   = 1 - TR;
c_root = (sigma_avg * pi * RT_diskR_I) / (Nb * (1 - t_c/2));

== matlab function RT_BladeElementForces/MATLAB Function7 ==
  data: c_root input; chord output; NondimRadialDis input; t_c input
function chord = fcn(c_root,  NondimRadialDis, t_c)

chord = c_root .* (1 - t_c .* NondimRadialDis);

== matlab function RT_BladeElementForces/MATLAB Function8 ==
  data: RT_DistanceY_I input; NondimRadialDis output; RT_diskR_I input
function NondimRadialDis = fcn(RT_DistanceY_I, RT_diskR_I)

NondimRadialDis = RT_DistanceY_I ./ RT_diskR_I;

== matlab function RT_BladeElementForces/MATLAB Function9 ==
  data: y_mat output; RT_diskR_I input; RT_BEDistFromEffSta_A input
function y_mat = fcn(RT_diskR_I, RT_BEDistFromEffSta_A)
% Scale non-dimensional radius → dimensional radius
y_vec = RT_BEDistFromEffSta_A(:)' * RT_diskR_I;   % [1×N]

% Replicate for 4 blades
y_mat = repmat(y_vec, 4, 1);   % [4×N]
end
